simulink model "Pacemaker_A1_full_v2"  (R2022b)
settings: Solver=FixedStepAuto  StartTime=0.0  StopTime=10.0  FixedStep=1e-3  RelTol=1e-3  EnableMultiTasking=on
undefined symbols (not defined in the file): D0, D1, D10, D11, D12, D13, D2, D3, D4, D5, D6, D7, D8, D9, PTA0, PTA1, PTA2, PTB23, PTB9, PTC16, PTC17, PTC2, PTC3, PTC4, PTD0, PTD1, PTD2, PTD3
libraries: frdmk64flib x16
settings Model: ExtModeTrigDuration=5  Creator=27161  LastModifiedBy=hoang
settings SolverCC: AlgebraicLoopSolver=TrustRegion
settings OptimizationCC: EnhancedBackFolding=on  PassReuseOutputArgsAs=Individual arguments  ZeroExternalMemoryAtStartup=off  ZeroInternalMemoryAtStartup=off  MaxStackSize=64  OptimizeBlockOrder=speed  DifferentSizesBufferReuse=on  OptimizationCustomize=off  EfficientTunableParamExpr=on
settings DebuggingCC: ParameterTunabilityLossMsg=error  UnconnectedInputMsg=warning  UnconnectedOutputMsg=warning  UnconnectedLineMsg=warning  SFMachineParentedDataDiag=warning
settings HardwareCC: ProdBitPerPointer=32  ProdBitPerSizeT=32  ProdBitPerPtrDiffT=32  ProdLargestAtomicInteger=Long  ProdLargestAtomicFloat=Double  ProdWordSize=32  ProdHWDeviceType=ARM Compatible->ARM Cortex
settings ModelReferenceCC: EnableRefExpFcnMdlSchedulingChecks=on
settings SFSimCC: MATLABDynamicMemAlloc=off
settings RTWCC: Description=Embedded Coder  SystemTargetFile=ert.tlc  HardwareBoard=NXP FRDM-K64F  TLCOptions="-aInlineSetEventsForThisBaseRateFcn=TLC_FALSE -aSuppressMultiTaskScheduler=TLC_FALSE  -aRateBasedStepFcn=0"  TemplateMakefile=ert_default_tmf  Toolchain=GNU Tools for ARM Embedded Processors
settings CodeAppCC: ForceParamTrailComments=on  IgnoreCustomStorageClasses=off  OperatorAnnotations=on  SimulinkDataObjDesc=on  SFDataObjDesc=on  InsertBlockDesc=on

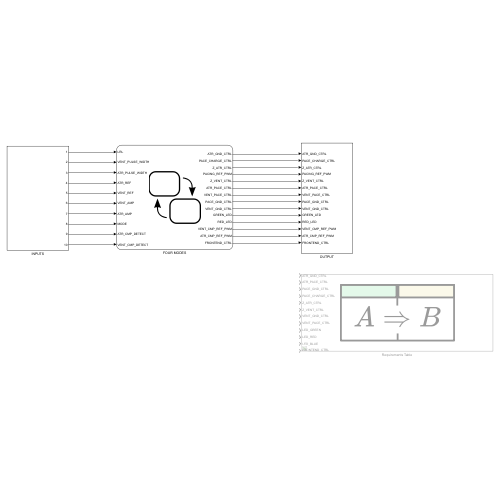
[thumbnail: Simulink's stored preview of the top-level diagram]
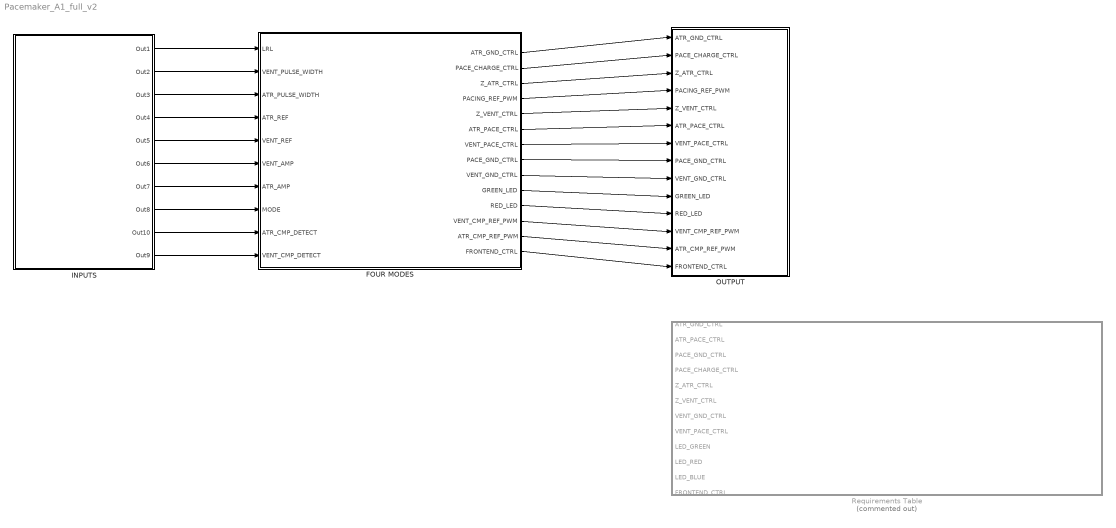
== system Pacemaker_A1_full_v2 ==
  FOUR MODES : Stateflow chart  TreatAsAtomicUnit=on
      settings: PortSchema="{\"entries\":[{\"content\":{\"sides\":[{\"content\":{\"connectorIds\":[\"In1\",\"In3\",\"In2\",\"In7\",\"In4\",\"In6\",\"In8\",\"In9\",\"In10\",\"In5\"]},\"type\":\"ConnectorPlacement.EquallySpacedRectSide\",\"uuid\":\"6661be6b-aedb-4592-878a-fd9116f5820d\"},{\"content\":{\"connectorIds\":[\"Out9\",\"Out1\",\"Out2\",\"Out3\",\"Out4\",\"Out5\",\"Out6\",\"Out8\",\"Out7\",\"Out11\",\"Out12\",\"Out13\",\"Out14\",\"Out10\"],\"side\":\"RIGHT\"},\"type\":\"ConnectorPlacement.EquallySpacedRectSide\",\"uuid\":\"f16586c3-0c99-4971-ba5f-75b93d25059c\"},{\"content\":{\"connectorIds\":[],\"side\":\"TOP\"},\"type\":\"ConnectorPlacement.EquallySpacedRectSide\",\"uuid\":\"27cb1bd0-c170-4ecc-a4df-3797e7aecef3\"}]},\"type\":\"ConnectorPlacement.EquallySpacedConnector\",\"uuid\":\"03557791-41f4-4916-8cde-1fcab0cf663d\"}],\"packageUris\":[\"http://schema.mathworks.com/mf0/Connector/R2020b\"],\"version\":\"1.0\"}"
  INPUTS : Subsystem
  OUTPUT : Subsystem
  Requirements Table : Requirements Table  Commented=on  TreatAsAtomicUnit=on
  wires:
  FOUR MODES/2(Z_ATR_CTRL) -> OUTPUT/3(Z_ATR_CTRL)
  FOUR MODES/9(ATR_GND_CTRL) -> OUTPUT/1(ATR_GND_CTRL)
  FOUR MODES/1(PACE_CHARGE_CTRL) -> OUTPUT/2(PACE_CHARGE_CTRL)
  FOUR MODES/3(PACING_REF_PWM) -> OUTPUT/4(PACING_REF_PWM)
  FOUR MODES/4(Z_VENT_CTRL) -> OUTPUT/5(Z_VENT_CTRL)
  FOUR MODES/5(ATR_PACE_CTRL) -> OUTPUT/6(ATR_PACE_CTRL)
  FOUR MODES/6(VENT_PACE_CTRL) -> OUTPUT/7(VENT_PACE_CTRL)
  FOUR MODES/7(VENT_GND_CTRL) -> OUTPUT/9(VENT_GND_CTRL)
  FOUR MODES/8(PACE_GND_CTRL) -> OUTPUT/8(PACE_GND_CTRL)
  INPUTS/1(Out1) -> FOUR MODES/1(LRL)
  INPUTS/2(Out2) -> FOUR MODES/3(VENT_PULSE_WIDTH)
  INPUTS/3(Out3) -> FOUR MODES/2(ATR_PULSE_WIDTH)
  INPUTS/4(Out4) -> FOUR MODES/7(ATR_REF)
  INPUTS/5(Out5) -> FOUR MODES/4(VENT_REF)
  INPUTS/6(Out6) -> FOUR MODES/6(VENT_AMP)
  INPUTS/8(Out8) -> FOUR MODES/9(MODE)
  INPUTS/7(Out7) -> FOUR MODES/8(ATR_AMP)
  FOUR MODES/11(GREEN_LED) -> OUTPUT/10(GREEN_LED)
  FOUR MODES/14(ATR_CMP_REF_PWM) -> OUTPUT/13(ATR_CMP_REF_PWM)
  FOUR MODES/13(VENT_CMP_REF_PWM) -> OUTPUT/12(VENT_CMP_REF_PWM)
  FOUR MODES/12(RED_LED) -> OUTPUT/11(RED_LED)
  FOUR MODES/10(FRONTEND_CTRL) -> OUTPUT/14(FRONTEND_CTRL)
  INPUTS/9(Out10) -> FOUR MODES/10(ATR_CMP_DETECT)
  INPUTS/10(Out9) -> FOUR MODES/5(VENT_CMP_DETECT)

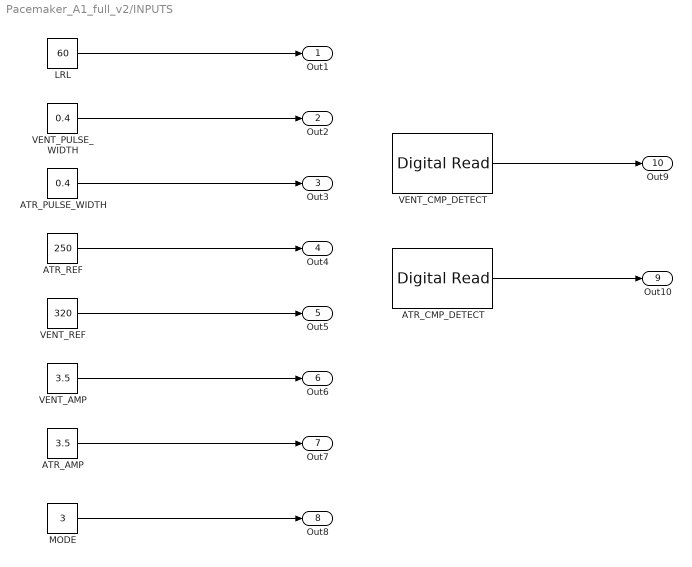
== system Pacemaker_A1_full_v2/INPUTS ==
  ATR_AMP : Constant  Value=3.5
  ATR_CMP_DETECT : frdmk64flib/Digital Read  Whichpin=PTC16 (D0)  SampleTime=-1
  ATR_PULSE_WIDTH : Constant  Value=0.4
  ATR_REF : Constant  Value=250
  LRL : Constant  Value=60
  MODE : Constant  Value=3
  VENT_AMP : Constant  Value=3.5
  VENT_CMP_DETECT : frdmk64flib/Digital Read  Whichpin=PTC17 (D1)  SampleTime=-1
  VENT_PULSE_WIDTH : Constant  Value=0.4
  VENT_REF : Constant  Value=320
  Out1 : Outport
  Out2 : Outport  Port=2
  Out3 : Outport  Port=3
  Out4 : Outport  Port=4
  Out5 : Outport  Port=5
  Out6 : Outport  Port=6
  Out7 : Outport  Port=7
  Out8 : Outport  Port=8
  Out10 : Outport  Port=9
  Out9 : Outport  Port=10
  wires:
  LRL/1 -> Out1/1
  VENT_PULSE_WIDTH/1 -> Out2/1
  ATR_PULSE_WIDTH/1 -> Out3/1
  ATR_REF/1 -> Out4/1
  VENT_REF/1 -> Out5/1
  VENT_AMP/1 -> Out6/1
  ATR_AMP/1 -> Out7/1
  MODE/1 -> Out8/1
  ATR_CMP_DETECT/1 -> Out10/1
  VENT_CMP_DETECT/1 -> Out9/1

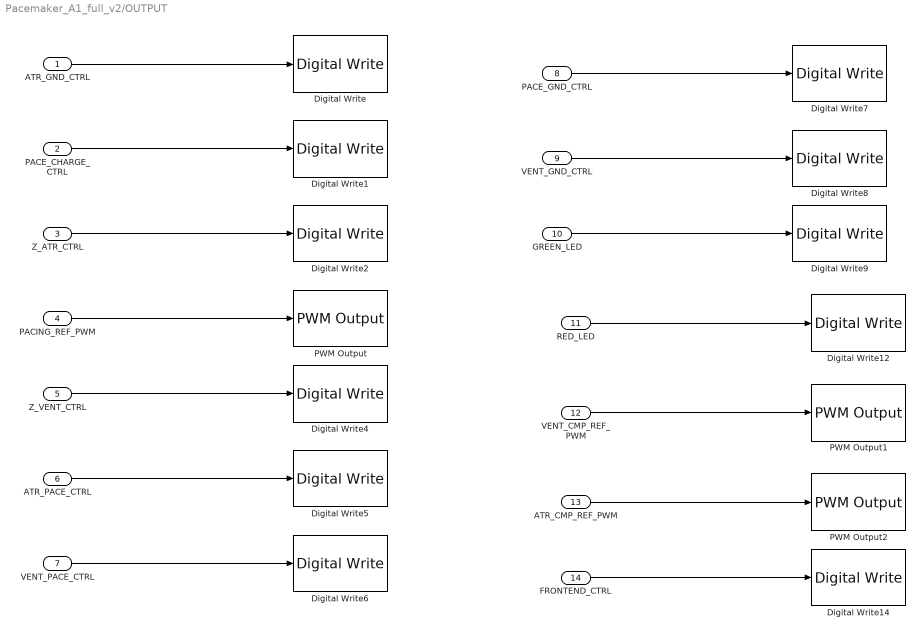
== system Pacemaker_A1_full_v2/OUTPUT ==
  ATR_GND_CTRL : Inport
  PACE_CHARGE_CTRL : Inport  Port=2
  Z_ATR_CTRL : Inport  Port=3
  PACING_REF_PWM : Inport  Port=4
  Z_VENT_CTRL : Inport  Port=5
  ATR_PACE_CTRL : Inport  Port=6
  VENT_PACE_CTRL : Inport  Port=7
  PACE_GND_CTRL : Inport  Port=8
  VENT_GND_CTRL : Inport  Port=9
  GREEN_LED : Inport  Port=10
  RED_LED : Inport  Port=11
  VENT_CMP_REF_PWM : Inport  Port=12
  ATR_CMP_REF_PWM : Inport  Port=13
  FRONTEND_CTRL : Inport  Port=14
  Digital Write : frdmk64flib/Digital Write  Whichpin=PTD2 (D11)
  Digital Write1 : frdmk64flib/Digital Write  Whichpin=PTB9 (D2)
  Digital Write12 : frdmk64flib/Digital Write  Whichpin=RED_LED
  Digital Write14 : frdmk64flib/Digital Write  Whichpin=PTD1 (D13)
  Digital Write2 : frdmk64flib/Digital Write  Whichpin=PTB23 (D4)
  Digital Write4 : frdmk64flib/Digital Write  Whichpin=PTC3 (D7)
  Digital Write5 : frdmk64flib/Digital Write  Whichpin=PTA0 (D8)
  Digital Write6 : frdmk64flib/Digital Write  Whichpin=PTC4 (D9)
  Digital Write7 : frdmk64flib/Digital Write  Whichpin=PTD0 (D10)
  Digital Write8 : frdmk64flib/Digital Write  Whichpin=PTD3 (D12)
  Digital Write9 : frdmk64flib/Digital Write  Whichpin=GREEN_LED
  PWM Output : frdmk64flib/PWM Output  Whichpin=PTA2 (D5)  InitialFrequency=2000  InitialDutyCycle=0
  PWM Output1 : frdmk64flib/PWM Output  Whichpin=PTA1 (D3)  InitialFrequency=2000  InitialDutyCycle=0
  PWM Output2 : frdmk64flib/PWM Output  Whichpin=PTC2 (D6)  InitialFrequency=2000  InitialDutyCycle=0
  wires:
  ATR_GND_CTRL/1 -> Digital Write/1
  PACE_CHARGE_CTRL/1 -> Digital Write1/1
  Z_ATR_CTRL/1 -> Digital Write2/1
  PACING_REF_PWM/1 -> PWM Output/1
  Z_VENT_CTRL/1 -> Digital Write4/1
  ATR_PACE_CTRL/1 -> Digital Write5/1
  VENT_PACE_CTRL/1 -> Digital Write6/1
  PACE_GND_CTRL/1 -> Digital Write7/1
  VENT_GND_CTRL/1 -> Digital Write8/1
  GREEN_LED/1 -> Digital Write9/1
  ATR_CMP_REF_PWM/1 -> PWM Output2/1
  VENT_CMP_REF_PWM/1 -> PWM Output1/1
  RED_LED/1 -> Digital Write12/1
  FRONTEND_CTRL/1 -> Digital Write14/1

== stateflow chart Pacemaker_A1_full_v2/Requirements Table ==
  (default) -> (junction 1073747182)
  (junction 1073747182) -> (junction 1073747183) : {
      | % SF_REQ_REV_07
      | }
  (junction 1073747183) -> (junction 1073747185) : {
      | % HEADER_ASSIGNMENTS
      |
      | }
  (junction 1073747185) -> (junction 1073747187) : {
      | % START_A_4
      | }
  (junction 1073747187) -> (junction 1073747189) : {
      | }
  (junction 1073747189) -> (junction 1073747191)
  (junction 1073747191) -> (junction 1073747193) : {
      | }
  (junction 1073747193) -> (junction 1073747195) : {
      | % END_A_4
      | }
  (junction 1073747195) -> (junction 1073747197) : {
      | % START_R_1
      | }
  (junction 1073747197) -> (junction 1073747199) : {
      | }
  (junction 1073747199) -> (junction 1073747201)
  (junction 1073747201) -> (junction 1073747203) [order 1] : [(((MODE) == (1)))]
  (junction 1073747201) -> (junction 1073747245) [order 2]
  (junction 1073747203) -> (junction 1073747205) : {
      |
      |
      | }
  (junction 1073747205) -> (junction 1073747207) : {
      | }
  (junction 1073747207) -> (junction 1073747209) : {
      | % START_R_7
      | }
  (junction 1073747209) -> (junction 1073747211) : {
      | }
  (junction 1073747211) -> (junction 1073747213)
  (junction 1073747213) -> (junction 1073747215) [order 1] : [duration((((prev(PACE_GND_CTRL)) == (true))) && (((prev(PACE_CHARGE_CTRL)) == (true))) && (((prev(ATR_GND_CTRL)) == (true))) && (((prev(ATR_PACE_CTRL)) == (false))) && (((prev(VENT_PACE_CTRL)) == (false))) && (((prev(VENT_GND_CTRL)) == (false))) && (((prev(Z_ATR_CTRL)) == (false))) && (((prev(Z_VENT_CTRL)) == (false))) && (((prev(LED_GREEN)) == (true)))) >= (60000/LRL - ATR_PULSE_WIDTH)/1000]
  (junction 1073747213) -> (junction 1073747221) [order 2]
  (junction 1073747215) -> (junction 1073747217) : {
      | reqtable_postcondition((((PACE_GND_CTRL) == (true))) && (((PACE_CHARGE_CTRL) == (false))) && (((ATR_GND_CTRL) == (false))) && (((ATR_PACE_CTRL) == (true))) && (((VENT_PACE_CTRL) == (false))) && (((VENT_GND_CTRL) == (false))) && (((Z_ATR_CTRL) == (false))) && (((Z_VENT_CTRL) == (false))) && (((LED_GREEN) == (false))), 'R:1.1');
      |
      |
      | }
  (junction 1073747217) -> (junction 1073747219) : {
      | }
  (junction 1073747219) -> (junction 1073747221)
  (junction 1073747221) -> (junction 1073747223)
  (junction 1073747223) -> (junction 1073747225) : {
      | % END_R_7
      | }
  (junction 1073747225) -> (junction 1073747227) : {
      | % START_R_34
      | }
  (junction 1073747227) -> (junction 1073747229) : {
      | }
  (junction 1073747229) -> (junction 1073747231)
  (junction 1073747231) -> (junction 1073747233) [order 1] : [duration((((prev(PACE_GND_CTRL)) == (true))) && (((prev(PACE_CHARGE_CTRL)) == (false))) && (((prev(ATR_GND_CTRL)) == (false))) && (((prev(ATR_PACE_CTRL)) == (true))) && (((prev(VENT_PACE_CTRL)) == (false))) && (((prev(VENT_GND_CTRL)) == (false))) && (((prev(Z_ATR_CTRL)) == (false))) && (((prev(Z_VENT_CTRL)) == (false))) && (((prev(LED_GREEN)) == (false)))) >= ATR_PULSE_WIDTH/1000]
  (junction 1073747231) -> (junction 1073747239) [order 2]
  (junction 1073747233) -> (junction 1073747235) : {
      | reqtable_postcondition((((PACE_GND_CTRL) == (true))) && (((PACE_CHARGE_CTRL) == (true))) && (((ATR_GND_CTRL) == (true))) && (((ATR_PACE_CTRL) == (false))) && (((VENT_PACE_CTRL) == (false))) && (((VENT_GND_CTRL) == (false))) && (((Z_ATR_CTRL) == (false))) && (((Z_VENT_CTRL) == (false))) && (((LED_GREEN) == (true))), 'R:1.2');
      |
      |
      | }
  (junction 1073747235) -> (junction 1073747237) : {
      | }
  (junction 1073747237) -> (junction 1073747239)
  (junction 1073747239) -> (junction 1073747241)
  (junction 1073747241) -> (junction 1073747243) : {
      | % END_R_34
      | }
  (junction 1073747243) -> (junction 1073747245)
  (junction 1073747245) -> (junction 1073747247)
  (junction 1073747247) -> (junction 1073747249) : {
      | % END_R_1
      | }
  (junction 1073747249) -> (junction 1073747251) : {
      | % START_R_10
      | }
  (junction 1073747251) -> (junction 1073747253) : {
      | }
  (junction 1073747253) -> (junction 1073747255)
  (junction 1073747255) -> (junction 1073747257) [order 1] : [(((MODE) == (2)))]
  (junction 1073747255) -> (junction 1073747299) [order 2]
  (junction 1073747257) -> (junction 1073747259) : {
      |
      |
      | }
  (junction 1073747259) -> (junction 1073747261) : {
      | }
  (junction 1073747261) -> (junction 1073747263) : {
      | % START_R_28
      | }
  (junction 1073747263) -> (junction 1073747265) : {
      | }
  (junction 1073747265) -> (junction 1073747267)
  (junction 1073747267) -> (junction 1073747269) [order 1] : [duration((((prev(PACE_GND_CTRL)) == (true))) && (((prev(PACE_CHARGE_CTRL)) == (true))) && (((prev(ATR_GND_CTRL)) == (false))) && (((prev(ATR_PACE_CTRL)) == (false))) && (((prev(VENT_PACE_CTRL)) == (false))) && (((prev(VENT_GND_CTRL)) == (true))) && (((prev(Z_ATR_CTRL)) == (false))) && (((prev(Z_VENT_CTRL)) == (false))) && (((prev(LED_RED)) == (true)))) >= (60000/LRL - VENT_PULSE_WIDTH)/1000]
  (junction 1073747267) -> (junction 1073747275) [order 2]
  (junction 1073747269) -> (junction 1073747271) : {
      | reqtable_postcondition((((PACE_GND_CTRL) == (true))) && (((PACE_CHARGE_CTRL) == (false))) && (((ATR_GND_CTRL) == (false))) && (((ATR_PACE_CTRL) == (false))) && (((VENT_PACE_CTRL) == (true))) && (((VENT_GND_CTRL) == (false))) && (((Z_ATR_CTRL) == (false))) && (((Z_VENT_CTRL) == (false))) && (((LED_RED) == (false))), 'R:2.1');
      |
      |
      | }
  (junction 1073747271) -> (junction 1073747273) : {
      | }
  (junction 1073747273) -> (junction 1073747275)
  (junction 1073747275) -> (junction 1073747277)
  (junction 1073747277) -> (junction 1073747279) : {
      | % END_R_28
      | }
  (junction 1073747279) -> (junction 1073747281) : {
      | % START_R_31
      | }
  (junction 1073747281) -> (junction 1073747283) : {
      | }
  (junction 1073747283) -> (junction 1073747285)
  (junction 1073747285) -> (junction 1073747287) [order 1] : [duration((((prev(PACE_GND_CTRL)) == (true))) && (((prev(PACE_CHARGE_CTRL)) == (false))) && (((prev(ATR_GND_CTRL)) == (false))) && (((prev(ATR_PACE_CTRL)) == (false))) && (((prev(VENT_PACE_CTRL)) == (true))) && (((prev(VENT_GND_CTRL)) == (false))) && (((prev(Z_ATR_CTRL)) == (false))) && (((prev(Z_VENT_CTRL)) == (false))) && (((prev(LED_RED)) == (false)))) >= VENT_PULSE_WIDTH/1000]
  (junction 1073747285) -> (junction 1073747293) [order 2]
  (junction 1073747287) -> (junction 1073747289) : {
      | reqtable_postcondition((((PACE_GND_CTRL) == (false))) && (((PACE_CHARGE_CTRL) == (true))) && (((ATR_GND_CTRL) == (false))) && (((ATR_PACE_CTRL) == (false))) && (((VENT_PACE_CTRL) == (false))) && (((VENT_GND_CTRL) == (true))) && (((Z_ATR_CTRL) == (false))) && (((Z_VENT_CTRL) == (false))) && (((LED_RED) == (true))), 'R:2.2');
      |
      |
      | }
  (junction 1073747289) -> (junction 1073747291) : {
      | }
  (junction 1073747291) -> (junction 1073747293)
  (junction 1073747293) -> (junction 1073747295)
  (junction 1073747295) -> (junction 1073747297) : {
      | % END_R_31
      | }
  (junction 1073747297) -> (junction 1073747299)
  (junction 1073747299) -> (junction 1073747301)
  (junction 1073747301) -> (junction 1073747303) : {
      | % END_R_10
      | }
  (junction 1073747303) -> (junction 1073747305) : {
      | % START_R_13
      | }
  (junction 1073747305) -> (junction 1073747307) : {
      | }
  (junction 1073747307) -> (junction 1073747309)
  (junction 1073747309) -> (junction 1073747311) [order 1] : [(((MODE) == (3)))]
  (junction 1073747309) -> (junction 1073747389) [order 2]
  (junction 1073747311) -> (junction 1073747313) : {
      |
      |
      | }
  (junction 1073747313) -> (junction 1073747315) : {
      | }
  (junction 1073747315) -> (junction 1073747317) : {
      | % START_R_19
      | }
  (junction 1073747317) -> (junction 1073747319) : {
      | }
  (junction 1073747319) -> (junction 1073747321)
  (junction 1073747321) -> (junction 1073747323) [order 1] : [duration((((prev(PACE_GND_CTRL)) == (true))) && (((prev(PACE_CHARGE_CTRL)) == (false))) && (((prev(ATR_GND_CTRL)) == (false))) && (((prev(ATR_PACE_CTRL)) == (false))) && (((prev(VENT_PACE_CTRL)) == (false))) && (((prev(VENT_GND_CTRL)) == (true))) && (((prev(Z_ATR_CTRL)) == (false))) && (((prev(Z_VENT_CTRL)) == (false))) && (((prev(LED_GREEN)) == (false))) && (((prev(FRONTEND_CTRL)) == (false)))) >= VENT_REF/1000]
  (junction 1073747321) -> (junction 1073747329) [order 2]
  (junction 1073747323) -> (junction 1073747325) : {
      | reqtable_postcondition((((PACE_GND_CTRL) == (true))) && (((PACE_CHARGE_CTRL) == (true))) && (((ATR_GND_CTRL) == (false))) && (((ATR_PACE_CTRL) == (false))) && (((VENT_PACE_CTRL) == (false))) && (((VENT_GND_CTRL) == (true))) && (((Z_ATR_CTRL) == (false))) && (((Z_VENT_CTRL) == (false))) && (((LED_RED) == (true))) && (((FRONTEND_CTRL) == (true))), 'R:3.1');
      |
      |
      | }
  (junction 1073747325) -> (junction 1073747327) : {
      | }
  (junction 1073747327) -> (junction 1073747329)
  (junction 1073747329) -> (junction 1073747331)
  (junction 1073747331) -> (junction 1073747333) : {
      | % END_R_19
      | }
  (junction 1073747333) -> (junction 1073747335) : {
      | % START_R_22
      | }
  (junction 1073747335) -> (junction 1073747337) : {
      | }
  (junction 1073747337) -> (junction 1073747339)
  (junction 1073747339) -> (junction 1073747341) [order 1] : [duration((((prev(PACE_GND_CTRL)) == (true))) && (((prev(PACE_CHARGE_CTRL)) == (true))) && (((prev(ATR_GND_CTRL)) == (false))) && (((prev(ATR_PACE_CTRL)) == (false))) && (((prev(VENT_PACE_CTRL)) == (false))) && (((prev(VENT_GND_CTRL)) == (true))) && (((prev(Z_ATR_CTRL)) == (false))) && (((prev(Z_VENT_CTRL)) == (false))) && (((prev(LED_RED)) == (true))) && (((prev(FRONTEND_CTRL)) == (true)))) >= (60000/LRL - VENT_PULSE_WIDTH-VENT_REF)/1000]
  (junction 1073747339) -> (junction 1073747347) [order 2]
  (junction 1073747341) -> (junction 1073747343) : {
      | reqtable_postcondition((((PACE_GND_CTRL) == (true))) && (((PACE_CHARGE_CTRL) == (false))) && (((ATR_GND_CTRL) == (false))) && (((ATR_PACE_CTRL) == (false))) && (((VENT_PACE_CTRL) == (true))) && (((VENT_GND_CTRL) == (false))) && (((Z_ATR_CTRL) == (false))) && (((Z_VENT_CTRL) == (false))) && (((LED_GREEN) == (true))), 'R:3.2');
      |
      |
      | }
  (junction 1073747343) -> (junction 1073747345) : {
      | }
  (junction 1073747345) -> (junction 1073747347)
  (junction 1073747347) -> (junction 1073747349)
  (junction 1073747349) -> (junction 1073747351) : {
      | % END_R_22
      | }
  (junction 1073747351) -> (junction 1073747353) : {
      | % START_R_43
      | }
  (junction 1073747353) -> (junction 1073747355) : {
      | }
  (junction 1073747355) -> (junction 1073747357)
  (junction 1073747357) -> (junction 1073747359) [order 1] : [duration((((prev(PACE_GND_CTRL)) == (true))) && (((prev(PACE_CHARGE_CTRL)) == (false))) && (((prev(ATR_GND_CTRL)) == (false))) && (((prev(ATR_PACE_CTRL)) == (false))) && (((prev(VENT_PACE_CTRL)) == (true))) && (((prev(VENT_GND_CTRL)) == (false))) && (((prev(Z_ATR_CTRL)) == (false))) && (((prev(Z_VENT_CTRL)) == (false))) && (((prev(LED_GREEN)) == (true)))) >= VENT_PULSE_WIDTH/1000]
  (junction 1073747357) -> (junction 1073747365) [order 2]
  (junction 1073747359) -> (junction 1073747361) : {
      | reqtable_postcondition((((PACE_GND_CTRL) == (true))) && (((PACE_CHARGE_CTRL) == (false))) && (((ATR_GND_CTRL) == (false))) && (((ATR_PACE_CTRL) == (false))) && (((VENT_PACE_CTRL) == (false))) && (((VENT_GND_CTRL) == (true))) && (((Z_ATR_CTRL) == (false))) && (((Z_VENT_CTRL) == (false))) && (((LED_RED) == (false))) && (((FRONTEND_CTRL) == (true))), 'R:3.3');
      |
      |
      | }
  (junction 1073747361) -> (junction 1073747363) : {
      | }
  (junction 1073747363) -> (junction 1073747365)
  (junction 1073747365) -> (junction 1073747367)
  (junction 1073747367) -> (junction 1073747369) : {
      | % END_R_43
      | }
  (junction 1073747369) -> (junction 1073747371) : {
      | % START_R_49
      | }
  (junction 1073747371) -> (junction 1073747373) : {
      | }
  (junction 1073747373) -> (junction 1073747375)
  (junction 1073747375) -> (junction 1073747377) [order 1] : [(((prev(PACE_GND_CTRL)) == (true))) && (((prev(PACE_CHARGE_CTRL)) == (true))) && (((prev(ATR_GND_CTRL)) == (false))) && (((prev(ATR_PACE_CTRL)) == (false))) && (((prev(VENT_PACE_CTRL)) == (false))) && (((prev(VENT_GND_CTRL)) == (true))) && (((prev(Z_ATR_CTRL)) == (false))) && (((prev(Z_VENT_CTRL)) == (false))) && (((prev(LED_RED)) == (true))) && (((prev(FRONTEND_CTRL)) == (true)))]
  (junction 1073747375) -> (junction 1073747383) [order 2]
  (junction 1073747377) -> (junction 1073747379) : {
      | reqtable_postcondition((((PACE_GND_CTRL) == (true))) && (((PACE_CHARGE_CTRL) == (false))) && (((ATR_GND_CTRL) == (false))) && (((ATR_PACE_CTRL) == (false))) && (((VENT_PACE_CTRL) == (false))) && (((VENT_GND_CTRL) == (true))) && (((Z_ATR_CTRL) == (false))) && (((Z_VENT_CTRL) == (false))) && (((LED_RED) == (false))) && (((FRONTEND_CTRL) == (false))), 'R:3.4');
      |
      |
      | }
  (junction 1073747379) -> (junction 1073747381) : {
      | }
  (junction 1073747381) -> (junction 1073747383)
  (junction 1073747383) -> (junction 1073747385)
  (junction 1073747385) -> (junction 1073747387) : {
      | % END_R_49
      | }
  (junction 1073747387) -> (junction 1073747389)
  (junction 1073747389) -> (junction 1073747391)
  (junction 1073747391) -> (junction 1073747393) : {
      | % END_R_13
      | }
  (junction 1073747393) -> (junction 1073747395) : {
      | % START_R_16
      | }
  (junction 1073747395) -> (junction 1073747397) : {
      | }
  (junction 1073747397) -> (junction 1073747399)
  (junction 1073747399) -> (junction 1073747401) [order 1] : [(((MODE) == (4)))]
  (junction 1073747399) -> (junction 1073747471) [order 2]
  (junction 1073747401) -> (junction 1073747403) : {
      |
      |
      | }
  (junction 1073747403) -> (junction 1073747405) : {
      | }
  (junction 1073747405) -> (junction 1073747407) : {
      | % START_R_37
      | }
  (junction 1073747407) -> (junction 1073747409) : {
      | }
  (junction 1073747409) -> (junction 1073747411)
  (junction 1073747411) -> (junction 1073747413) [order 1] : [duration((((prev(PACE_GND_CTRL)) == (true))) && (((prev(PACE_CHARGE_CTRL)) == (false))) && (((prev(ATR_GND_CTRL)) == (true))) && (((prev(ATR_PACE_CTRL)) == (false))) && (((prev(VENT_PACE_CTRL)) == (false))) && (((prev(VENT_GND_CTRL)) == (false))) && (((prev(Z_ATR_CTRL)) == (false))) && (((prev(Z_VENT_CTRL)) == (false))) && (((prev(LED_GREEN)) == (false))) && (((prev(FRONTEND_CTRL)) == (false)))) >= ATR_REF/1000]
  (junction 1073747411) -> (junction 1073747419) [order 2]
  (junction 1073747413) -> (junction 1073747415) : {
      | reqtable_postcondition((((PACE_GND_CTRL) == (true))) && (((PACE_CHARGE_CTRL) == (true))) && (((ATR_GND_CTRL) == (true))) && (((ATR_PACE_CTRL) == (false))) && (((VENT_PACE_CTRL) == (false))) && (((VENT_GND_CTRL) == (false))) && (((Z_ATR_CTRL) == (false))) && (((Z_VENT_CTRL) == (false))) && (((LED_GREEN) == (true))) && (((FRONTEND_CTRL) == (true))), 'R:4.1');
      |
      |
      | }
  (junction 1073747415) -> (junction 1073747417) : {
      | }
  (junction 1073747417) -> (junction 1073747419)
  (junction 1073747419) -> (junction 1073747421)
  (junction 1073747421) -> (junction 1073747423) : {
      | % END_R_37
      | }
  (junction 1073747423) -> (junction 1073747425) : {
      | % START_R_40
      | }
  (junction 1073747425) -> (junction 1073747427) : {
      | }
  (junction 1073747427) -> (junction 1073747429)
  (junction 1073747429) -> (junction 1073747431) [order 1] : [duration((((prev(PACE_GND_CTRL)) == (true))) && (((prev(PACE_CHARGE_CTRL)) == (true))) && (((prev(ATR_GND_CTRL)) == (true))) && (((prev(ATR_PACE_CTRL)) == (false))) && (((prev(VENT_PACE_CTRL)) == (false))) && (((prev(VENT_GND_CTRL)) == (false))) && (((prev(Z_ATR_CTRL)) == (false))) && (((prev(Z_VENT_CTRL)) == (false))) && (((prev(LED_GREEN)) == (true))) && (((prev(FRONTEND_CTRL)) == (true)))) >= (60000/LRL - ATR_PULSE_WIDTH-ATR_REF)/1000]
  (junction 1073747429) -> (junction 1073747437) [order 2]
  (junction 1073747431) -> (junction 1073747433) : {
      | reqtable_postcondition((((PACE_GND_CTRL) == (true))) && (((PACE_CHARGE_CTRL) == (false))) && (((ATR_GND_CTRL) == (false))) && (((ATR_PACE_CTRL) == (true))) && (((VENT_PACE_CTRL) == (false))) && (((VENT_GND_CTRL) == (false))) && (((Z_ATR_CTRL) == (false))) && (((Z_VENT_CTRL) == (false))) && (((LED_RED) == (true))), 'R:4.2');
      |
      |
      | }
  (junction 1073747433) -> (junction 1073747435) : {
      | }
  (junction 1073747435) -> (junction 1073747437)
  (junction 1073747437) -> (junction 1073747439)
  (junction 1073747439) -> (junction 1073747441) : {
      | % END_R_40
      | }
  (junction 1073747441) -> (junction 1073747443) : {
      | % START_R_46
      | }
  (junction 1073747443) -> (junction 1073747445) : {
      | }
  (junction 1073747445) -> (junction 1073747447)
  (junction 1073747447) -> (junction 1073747449) [order 1] : [duration((((prev(PACE_GND_CTRL)) == (true))) && (((prev(PACE_CHARGE_CTRL)) == (false))) && (((prev(ATR_GND_CTRL)) == (false))) && (((prev(ATR_PACE_CTRL)) == (true))) && (((prev(VENT_PACE_CTRL)) == (false))) && (((prev(VENT_GND_CTRL)) == (false))) && (((prev(Z_ATR_CTRL)) == (false))) && (((prev(Z_VENT_CTRL)) == (false))) && (((prev(LED_RED)) == (true)))) >= ATR_PULSE_WIDTH/1000]
  (junction 1073747447) -> (junction 1073747455) [order 2]
  (junction 1073747449) -> (junction 1073747451) : {
      | reqtable_postcondition((((PACE_GND_CTRL) == (true))) && (((PACE_CHARGE_CTRL) == (false))) && (((ATR_GND_CTRL) == (true))) && (((ATR_PACE_CTRL) == (false))) && (((VENT_PACE_CTRL) == (false))) && (((VENT_GND_CTRL) == (false))) && (((Z_ATR_CTRL) == (false))) && (((Z_VENT_CTRL) == (false))) && (((LED_GREEN) == (false))) && (((FRONTEND_CTRL) == (true))), 'R:4.3');
      |
      |
      | }
  (junction 1073747451) -> (junction 1073747453) : {
      | }
  (junction 1073747453) -> (junction 1073747455)
  (junction 1073747455) -> (junction 1073747457)
  (junction 1073747457) -> (junction 1073747459) : {
      | % END_R_46
      | }
  (junction 1073747459) -> (junction 1073747494) : {
      | % START_R_52
      | }
  (junction 1073747494) -> (junction 1073747496) : {
      | }
  (junction 1073747496) -> (junction 1073747498)
  (junction 1073747498) -> (junction 1073747500) [order 1] : [(((prev(PACE_GND_CTRL)) == (true))) && (((prev(PACE_CHARGE_CTRL)) == (true))) && (((prev(ATR_GND_CTRL)) == (true))) && (((prev(ATR_PACE_CTRL)) == (false))) && (((prev(VENT_PACE_CTRL)) == (false))) && (((prev(VENT_GND_CTRL)) == (false))) && (((prev(Z_ATR_CTRL)) == (false))) && (((prev(Z_VENT_CTRL)) == (false))) && (((prev(LED_GREEN)) == (true))) && (((prev(FRONTEND_CTRL)) == (true)))]
  (junction 1073747498) -> (junction 1073747506) [order 2]
  (junction 1073747500) -> (junction 1073747502) : {
      | reqtable_postcondition((((PACE_GND_CTRL) == (true))) && (((PACE_CHARGE_CTRL) == (false))) && (((ATR_GND_CTRL) == (true))) && (((ATR_PACE_CTRL) == (false))) && (((VENT_PACE_CTRL) == (false))) && (((VENT_GND_CTRL) == (false))) && (((Z_ATR_CTRL) == (false))) && (((Z_VENT_CTRL) == (false))) && (((LED_GREEN) == (false))) && (((FRONTEND_CTRL) == (false))), 'R:4.4');
      |
      |
      | }
  (junction 1073747502) -> (junction 1073747504) : {
      | }
  (junction 1073747504) -> (junction 1073747506)
  (junction 1073747506) -> (junction 1073747508)
  (junction 1073747508) -> (junction 1073747510) : {
      | % END_R_52
      | }
  (junction 1073747510) -> (junction 1073747471)
  (junction 1073747471) -> (junction 1073747473)
  (junction 1073747473) -> (junction 1073747475) : {
      | % END_R_16
      | }
  data: ATR_GND_CTRL input; ATR_PACE_CTRL input; PACE_GND_CTRL input; PACE_CHARGE_CTRL input; Z_ATR_CTRL input; Z_VENT_CTRL input; VENT_GND_CTRL input; VENT_PACE_CTRL input; LED_GREEN input; LED_RED input; LED_BLUE input; FRONTEND_CTRL input

== stateflow chart Pacemaker_A1_full_v2/FOUR MODES ==
  note: In the pacing state, we connect C22 to C21 to pace the Atrium.
  note: In the AOO initial state, we start charging C22 to prepare to pace.
      | Also, we begin to discharge C21 from the last pace.
  state AOO_PACING
    PACE_CHARGE_CTRL = false;
    PACE_GND_CTRL = true;
    ATR_PACE_CTRL = true;
    ATR_GND_CTRL = false;
    Z_ATR_CTRL = false;
    Z_VENT_CTRL = false;
    VENT_GND_CTRL = false;
    VENT_PACE_CTRL = false;
    GREEN_LED =0;
  state AOO_INITIAL
    entry:
    ATR_PACE_CTRL = false;
    ATR_GND_CTRL = true;
    VENT_GND_CTRL = false;
    VENT_PACE_CTRL = false;
    PACE_CHARGE_CTRL = true;
    PACE_GND_CTRL = true;
    Z_ATR_CTRL = false;
    Z_VENT_CTRL = false;
    PACING_REF_PWM = ATR_AMP*20
    GREEN_LED = 1;
  note: We have a total cycle of 60s/LRL(BPM)
  note: In the MainState, we set all of our set points to 0 and detect which mode we go next.
  state MainState
    entry:
    ATR_PACE_CTRL = false;
    ATR_GND_CTRL = false;
    VENT_GND_CTRL = false;
    VENT_PACE_CTRL = false;
    PACE_CHARGE_CTRL = false;
    PACE_GND_CTRL = false;
    Z_ATR_CTRL = false;
    Z_VENT_CTRL = false;
    FRONTEND_CTRL = false;
  note: In the pacing state, we connect C22 to C21 to pace the Atrium
  note: In the VOO initial state, we start charging C22 to prepare to pace.
      | Also, we begin to discharge C21 from the last pace.
  state VOO_INITIAL
    entry:
    ATR_PACE_CTRL = false;
    ATR_GND_CTRL = false;
    VENT_GND_CTRL = true;
    VENT_PACE_CTRL = false;
    PACE_CHARGE_CTRL = true;
    PACE_GND_CTRL = true;
    Z_ATR_CTRL = false;
    Z_VENT_CTRL = false;
    PACING_REF_PWM = VENT_AMP*20
    RED_LED = 1;
  note: We have a total cycle of 60s/LRL(BPM)
  state VOO_PACING
    PACE_CHARGE_CTRL = false;
    PACE_GND_CTRL = true;
    ATR_PACE_CTRL = false;
    ATR_GND_CTRL = false;
    Z_ATR_CTRL = false;
    Z_VENT_CTRL = false;
    VENT_GND_CTRL = false;
    VENT_PACE_CTRL = true;
    RED_LED =0;
  note: In the initial state of AAI, we have
      | sensor on to detact if the input voltage is higher
      | than our set threshlod.
      |
      | We also charge C22 for possible pacing
      | state happen when not detection of natural
      | pulse, and discharge C21 to end the pacing state.
      |
      | LED light is off at initial state.
  state AAI_INITIAL
    entry:
    FRONTEND_CTRL= true;
    ATR_PACE_CTRL = false;
    VENT_PACE_CTRL = false;
    PACING_REF_PWM = ATR_AMP*20;
    PACE_CHARGE_CTRL = true;
    Z_ATR_CTRL = false;
    Z_VENT_CTRL = false;
    PACE_GND_CTRL = true;
    VENT_GND_CTRL = false;
    ATR_GND_CTRL = true;
    ATR_CMP_REF_PWM = ATR_AMP*20;
    GREEN_LED = 1;
  note: After a pulse width, stop pacing
  note: When no detect natural pulse, pace the atrium
      | with connecting C22 to C11. Then wait for 1 cycle.
  state AAI_PACING
    entry:
    PACE_CHARGE_CTRL = false;
    PACE_GND_CTRL = true;
    ATR_PACE_CTRL = true;
    ATR_GND_CTRL = false;
    Z_ATR_CTRL = false;
    Z_VENT_CTRL = false;
    VENT_GND_CTRL = false;
    VENT_PACE_CTRL = false;
    RED_LED = 1;
  note: In the Refractory state, sensor turn off.
      | A signal of this happen will have red LED turn on.
      | After a refractory period, go back to initial state.
  state VVI_REF
    entry:
    FRONTEND_CTRL = true;
    VENT_PACE_CTRL = false;
    VENT_GND_CTRL = true;
    PACING_REF_PWM = VENT_AMP*20;
    PACE_CHARGE_CTRL = false;
    PACE_GND_CTRL = true;
    RED_LED = 0;
  state AAI_REF
    entry:
    FRONTEND_CTRL = true;
    ATR_PACE_CTRL = false;
    ATR_GND_CTRL = true;
    ATR_CMP_REF_PWM = ATR_AMP*20;
    PACE_CHARGE_CTRL = false;
    PACE_GND_CTRL = true;
    GREEN_LED = 0;
  state VVI_INITIAL
    entry:
    Z_ATR_CTRL = false;
    Z_VENT_CTRL = false;
    PACING_REF_PWM = VENT_AMP*20;
    PACE_GND_CTRL = true;
    VENT_GND_CTRL = true;
    ATR_GND_CTRL = false;
    ATR_PACE_CTRL = false;
    VENT_PACE_CTRL = false;
    PACE_CHARGE_CTRL = true;
    VENT_CMP_REF_PWM = VENT_AMP*20;
    FRONTEND_CTRL= true;
    RED_LED = 1;
  note: In the initial state of VVI, we turn the
      | sensor on to detect if the input voltage is higher
      | than our set threshlod.
      |
      | We also charge C22 for possible pacing
      | state happen when not detection of natural
      | pulse, and discharge C21 to end the pacing state.
      |
      | LED light is off at initial state.
  note: In the Refractory state, sensor turn off.
      | A signal of this happen will have red LED turn on.
      | After a refractory period, go back to initial state.
  state VVI_PACING
    entry:
    PACE_CHARGE_CTRL = false;
    PACE_GND_CTRL = true;
    ATR_PACE_CTRL = false;
    ATR_GND_CTRL = false;
    Z_ATR_CTRL = false;
    Z_VENT_CTRL = false;
    VENT_GND_CTRL = false;
    VENT_PACE_CTRL = true;
    GREEN_LED = 1;
  note: Discharging C22 to C21 to pace the ventricle.
      | Same as VOO pacing.
  AOO_INITIAL -> AOO_PACING : [after(60000/LRL - ATR_PULSE_WIDTH,msec)]
  (default) -> MainState [order 1]
  MainState -> AOO_INITIAL [order 1] : [MODE == 1]
  AOO_PACING -> AOO_INITIAL : [after(ATR_PULSE_WIDTH,msec)]
  (default) -> AAI_INITIAL [order 2]
  MainState -> AAI_INITIAL [order 4] : [MODE == 4]
  VOO_INITIAL -> VOO_PACING : [after(60000/LRL - VENT_PULSE_WIDTH,msec)]
  MainState -> VOO_INITIAL [order 2] : [MODE == 2]
  VOO_PACING -> VOO_INITIAL : [after(VENT_PULSE_WIDTH,msec)]
  MainState -> VVI_INITIAL [order 3] : [MODE == 3]
  AAI_INITIAL -> AAI_PACING [order 1] : [(ATR_CMP_DETECT == false) && after(60000/LRL - ATR_PULSE_WIDTH - ATR_REF,msec)]
  AAI_INITIAL -> AAI_REF [order 2] : [ATR_CMP_DETECT == true]
  AAI_REF -> AAI_INITIAL : [after(ATR_REF, msec)]
  VVI_REF -> VVI_INITIAL : [after(VENT_REF, msec)]
  AAI_PACING -> AAI_REF : [after(ATR_PULSE_WIDTH,msec)]
  VVI_INITIAL -> VVI_REF [order 2] : [VENT_CMP_DETECT == 1]
  VVI_PACING -> VVI_REF : [after(VENT_PULSE_WIDTH,msec)]
  VVI_INITIAL -> VVI_PACING [order 1] : [(VENT_CMP_DETECT == 0) && after(60000/LRL - VENT_PULSE_WIDTH - VENT_REF,msec)]
  data: PACE_CHARGE_CTRL output; Z_ATR_CTRL output; PACING_REF_PWM output; Z_VENT_CTRL output; ATR_PACE_CTRL output; VENT_PACE_CTRL output; VENT_GND_CTRL output; PACE_GND_CTRL output; ATR_GND_CTRL output; LRL input; ATR_PULSE_WIDTH input; VENT_PULSE_WIDTH input; FRONTEND_CTRL output; GREEN_LED output; VENT_REF input; VENT_CMP_DETECT input; VENT_AMP input; ATR_REF input; RED_LED output; ATR_AMP input; MODE input; VENT_CMP_REF_PWM output; ATR_CMP_DETECT input; ATR_CMP_REF_PWM output
